simulink model "robot_segway_bloques"  (R2023b)
settings: Solver=ode15s  StartTime=0.0  StopTime=tiempo_final  MaxStep=1e-3  RelTol=1e-5  AbsTol=1e-7
values from neighbouring files (symbols this model uses):
  par = parametros_simulink(P, C)    [cargar_workspace.m]    (also in construir_robot_bloques.m = -R f   (manual sec. 7)'; simular_ode.m)
  Ts = se.Ts    [robot_controlador.m]    (also in simular_ode.m = P.sens.Ts; simular_slx.m = P.sens.Ts)
undefined symbols (not defined in the file or in its folder): angulo_servo_inicial, encoders_iniciales, estados_iniciales, inclinacion_inicial_est, medidas_iniciales, retardo_muestras, semilla
libraries: simulink x10
(part 2 of 2)

== system robot_segway_bloques/Robot/Servo y pata ==
  note: Servo PD sobre theta(l) con limite par-velocidad, F_l = n_servos tau dtheta/dl ; topes de carrera ; flexor opcional en serie (l_mec) (manual sec. 5 y 8)
  comandos : Inport
  cuerpo : Inport  Port=2
  1 entre m mecanismo : Gain  Gain=1/par.pata.masa_mecanismo
  Flexor (resorte en serie) : Subsystem
  Servo (PD con limite par-velocidad) : Subsystem
  Topes de carrera : Subsystem
  acel mec (si flexor) : Switch  Criteria=u2 > Threshold  Threshold=0.5  SaturateOnIntegerOverflow=off  InputSameDT=off
  amortiguamiento de pata b_pata : Gain  Gain=par.cuerpo.amort_pata
  amortiguamiento del mecanismo : Gain  Gain=par.cuerpo.amort_pata
  bus pata : BusCreator  Inputs=5
  cero : Constant  Value=0
  consigna : BusSelector  OutputSignals=angulo_servo_ref
  d largo mec (si flexor) : Switch  Criteria=u2 > Threshold  Threshold=0.5  SaturateOnIntegerOverflow=off  InputSameDT=off
  flexor activo : Constant  Value=par.pata.flexor_activo
  fuerza sobre l : Switch  Criteria=u2 > Threshold  Threshold=0.5  SaturateOnIntegerOverflow=off  InputSameDT=off
  integrador largo mecanismo : Integrator  InitialCondition=estados_iniciales(19)
  integrador vel mecanismo : Integrator  InitialCondition=estados_iniciales(20)
  largo de pata : BusSelector  OutputSignals=largo_pata,d_largo_pata
  largo que mueve el servo : Switch  Criteria=u2 > Threshold  Threshold=0.5  SaturateOnIntegerOverflow=off  InputSameDT=off
  servo + topes - amort : Sum  Inputs=++-
  servo - flexor + topes - amort : Sum  Inputs=+-+-
  velocidad que ve el servo : Switch  Criteria=u2 > Threshold  Threshold=0.5  SaturateOnIntegerOverflow=off  InputSameDT=off
  pata : Outport
  wires:
  comandos/1 -> consigna/1
  cuerpo/1 -> largo de pata/1
  integrador vel mecanismo/1 -> d largo mec (si flexor)/1, velocidad que ve el servo/1, Flexor (resorte en serie)/3(d_largo_mecanismo), amortiguamiento del mecanismo/1, bus pata/5  "d_largo_mecanismo"
  flexor activo/1 -> d largo mec (si flexor)/2, acel mec (si flexor)/2, largo que mueve el servo/2, velocidad que ve el servo/2, fuerza sobre l/2
  cero/1 -> d largo mec (si flexor)/3, acel mec (si flexor)/3
  d largo mec (si flexor)/1 -> integrador largo mecanismo/1
  acel mec (si flexor)/1 -> integrador vel mecanismo/1
  integrador largo mecanismo/1 -> largo que mueve el servo/1, Flexor (resorte en serie)/1(largo_mecanismo), bus pata/4  "largo_mecanismo"
  largo de pata/1 -> largo que mueve el servo/3, Flexor (resorte en serie)/2(largo_pata)  "<largo_pata>"
  largo de pata/2 -> velocidad que ve el servo/3, Flexor (resorte en serie)/4(d_largo_pata), amortiguamiento de pata b_pata/1  "<d_largo_pata>"
  consigna/1 -> Servo (PD con limite par-velocidad)/1(angulo_ref)  "<angulo_servo_ref>"
  largo que mueve el servo/1 -> Servo (PD con limite par-velocidad)/2(largo), Topes de carrera/1(largo)  "largo_q"
  velocidad que ve el servo/1 -> Servo (PD con limite par-velocidad)/3(d_largo), Topes de carrera/2(d_largo)  "d_largo_q"
  Servo (PD con limite par-velocidad)/3(fuerza_servo) -> servo + topes - amort/1, servo - flexor + topes - amort/1  "fuerza_servo"
  Topes de carrera/1(fuerza_tope) -> servo + topes - amort/2, servo - flexor + topes - amort/3  "fuerza_topes"
  amortiguamiento de pata b_pata/1 -> servo + topes - amort/3
  Flexor (resorte en serie)/1(fuerza_flexor) -> fuerza sobre l/1, servo - flexor + topes - amort/2  "fuerza_flexor"
  servo + topes - amort/1 -> fuerza sobre l/3
  amortiguamiento del mecanismo/1 -> servo - flexor + topes - amort/4
  servo - flexor + topes - amort/1 -> 1 entre m mecanismo/1
  1 entre m mecanismo/1 -> acel mec (si flexor)/1
  fuerza sobre l/1 -> bus pata/1  "fuerza_pata"
  Servo (PD con limite par-velocidad)/1(par_servo) -> bus pata/2  "par_servo"
  Servo (PD con limite par-velocidad)/2(angulo_servo) -> bus pata/3  "angulo_servo"
  bus pata/1 -> pata/1

== system robot_segway_bloques/Sensores/Acelerometro ==
  f_x : Inport
  f_y : Inport  Port=2
  f_x + ruido : Sum
  f_y + ruido : Sum
  rms del ruido x : Gain  Gain=par.sensores.acel_ruido
  rms del ruido y : Gain  Gain=par.sensores.acel_ruido
  ruido eje x : RandomNumber  Seed=semilla+1  SampleTime=Ts
  ruido eje y : RandomNumber  Seed=semilla+2  SampleTime=Ts
  acel_x : Outport
  acel_y : Outport  Port=2
  wires:
  rms del ruido y/1 -> f_y + ruido/2
  ruido eje y/1 -> rms del ruido y/1
  ruido eje x/1 -> rms del ruido x/1
  f_y/1 -> f_y + ruido/1
  f_x/1 -> f_x + ruido/1
  f_y + ruido/1 -> acel_y/1
  f_x + ruido/1 -> acel_x/1
  rms del ruido x/1 -> f_x + ruido/2

== system robot_segway_bloques/Sensores/Encoders ==
  ang_izq : Inport
  ang_der : Inport  Port=2
  cuenta entera der : Rounding
  cuenta entera izq : Rounding
  cuentas por radian der : Gain  Gain=par.sensores.CPR/(2*pi)
  cuentas por radian izq : Gain  Gain=par.sensores.CPR/(2*pi)
  encoder habilitado : Constant  Value=par.sensores.encoder
  si hay encoder der : Switch  Criteria=u2 > Threshold  Threshold=0.5  SaturateOnIntegerOverflow=off  InputSameDT=off
  si hay encoder izq : Switch  Criteria=u2 > Threshold  Threshold=0.5  SaturateOnIntegerOverflow=off  InputSameDT=off
  sin encoder (NaN) : Constant  Value=NaN
  encoder_izq : Outport
  encoder_der : Outport  Port=2
  wires:
  cuentas por radian der/1 -> cuenta entera der/1
  cuenta entera der/1 -> si hay encoder der/1
  encoder habilitado/1 -> si hay encoder izq/2, si hay encoder der/2
  ang_izq/1 -> cuentas por radian izq/1
  cuenta entera izq/1 -> si hay encoder izq/1
  ang_der/1 -> cuentas por radian der/1
  cuentas por radian izq/1 -> cuenta entera izq/1
  si hay encoder der/1 -> encoder_der/1
  sin encoder (NaN)/1 -> si hay encoder izq/3, si hay encoder der/3
  si hay encoder izq/1 -> encoder_izq/1

== system robot_segway_bloques/Sensores/Giroscopio ==
  vel_cabeceo : Inport
  giro + sesgo + ruido : Sum  Inputs=+++
  rms del ruido : Gain  Gain=par.sensores.gyro_ruido
  ruido blanco : RandomNumber  Seed=semilla  SampleTime=Ts
  saturacion del giroscopo : Saturate  UpperLimit=par.sensores.gyro_sat  LowerLimit=-par.sensores.gyro_sat
  sesgo : Constant  Value=par.sensores.gyro_sesgo
  giroscopo : Outport
  wires:
  ruido blanco/1 -> rms del ruido/1
  giro + sesgo + ruido/1 -> saturacion del giroscopo/1
  vel_cabeceo/1 -> giro + sesgo + ruido/1
  sesgo/1 -> giro + sesgo + ruido/2
  saturacion del giroscopo/1 -> giroscopo/1
  rms del ruido/1 -> giro + sesgo + ruido/3  "ruido"

== system robot_segway_bloques/Robot/Contacto rueda-piso/Friccion rueda derecha ==
  deslizamiento : Inport
  normal_por_rueda : Inport  Port=2
  mu : Inport  Port=3
  contacto : Inport  Port=4
  1 entre v0 : Gain  Gain=1/par.rueda.v0
  Coulomb - viscosa : Sum  Inputs=+-
  mu N tanh : Product  Inputs=***
  solo con contacto : Product  Inputs=**
  tanh : Trigonometry  Operator=tanh
  viscosa c_v : Gain  Gain=par.rueda.c_v
  fuerza : Outport
  wires:
  deslizamiento/1 -> viscosa c_v/1, 1 entre v0/1
  Coulomb - viscosa/1 -> solo con contacto/1
  mu N tanh/1 -> Coulomb - viscosa/1
  tanh/1 -> mu N tanh/3
  normal_por_rueda/1 -> mu N tanh/2
  1 entre v0/1 -> tanh/1
  mu/1 -> mu N tanh/1
  viscosa c_v/1 -> Coulomb - viscosa/2
  contacto/1 -> solo con contacto/2
  solo con contacto/1 -> fuerza/1

== system robot_segway_bloques/Robot/Contacto rueda-piso/Friccion rueda izquierda ==
  deslizamiento : Inport
  normal_por_rueda : Inport  Port=2
  mu : Inport  Port=3
  contacto : Inport  Port=4
  1 entre v0 : Gain  Gain=1/par.rueda.v0
  Coulomb - viscosa : Sum  Inputs=+-
  mu N tanh : Product  Inputs=***
  solo con contacto : Product  Inputs=**
  tanh : Trigonometry  Operator=tanh
  viscosa c_v : Gain  Gain=par.rueda.c_v
  fuerza : Outport
  wires:
  Coulomb - viscosa/1 -> solo con contacto/1
  mu/1 -> mu N tanh/1
  deslizamiento/1 -> viscosa c_v/1, 1 entre v0/1
  normal_por_rueda/1 -> mu N tanh/2
  1 entre v0/1 -> tanh/1
  tanh/1 -> mu N tanh/3
  mu N tanh/1 -> Coulomb - viscosa/1
  viscosa c_v/1 -> Coulomb - viscosa/2
  contacto/1 -> solo con contacto/2
  solo con contacto/1 -> fuerza/1

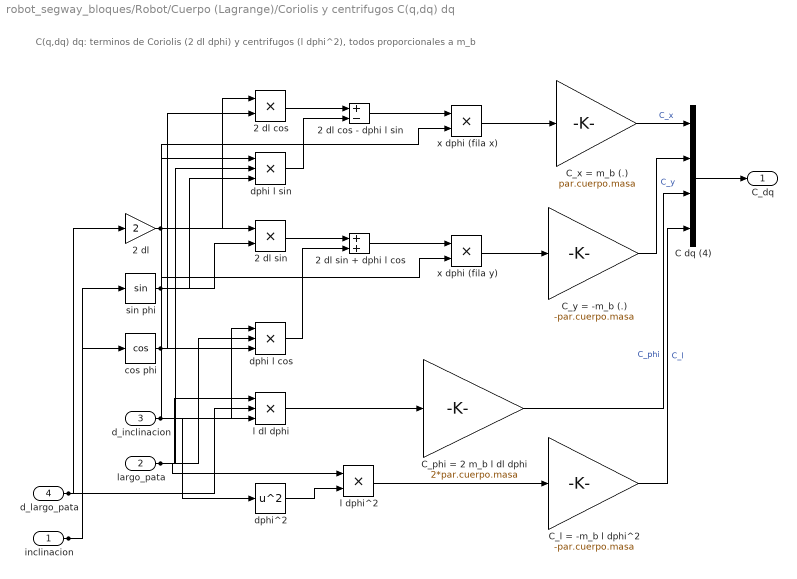
== system robot_segway_bloques/Robot/Cuerpo (Lagrange)/Coriolis y centrifugos C(q,dq) dq ==
  note: C(q,dq) dq: terminos de Coriolis (2 dl dphi) y centrifugos (l dphi^2), todos proporcionales a m_b
  inclinacion : Inport
  largo_pata : Inport  Port=2
  d_inclinacion : Inport  Port=3
  d_largo_pata : Inport  Port=4
  2 dl : Gain  Gain=2
  2 dl cos : Product  Inputs=**
  2 dl cos - dphi l sin : Sum  Inputs=+-
  2 dl sin : Product  Inputs=**
  2 dl sin + dphi l cos : Sum
  C dq (4) : Mux
  C_l = -m_b l dphi^2 : Gain  Gain=-par.cuerpo.masa
  C_phi = 2 m_b l dl dphi : Gain  Gain=2*par.cuerpo.masa
  C_x = m_b (.) : Gain  Gain=par.cuerpo.masa
  C_y = -m_b (.) : Gain  Gain=-par.cuerpo.masa
  cos phi : Trigonometry  Operator=cos
  dphi l cos : Product  Inputs=***
  dphi l sin : Product  Inputs=***
  dphi^2 : Math  Operator=square
  l dl dphi : Product  Inputs=***
  l dphi^2 : Product  Inputs=**
  sin phi : Trigonometry
  x dphi (fila x) : Product  Inputs=**
  x dphi (fila y) : Product  Inputs=**
  C_dq : Outport
  wires:
  largo_pata/1 -> l dphi^2/1, dphi l cos/2, dphi l sin/2, l dl dphi/1
  2 dl/1 -> 2 dl cos/1, 2 dl sin/1
  d_largo_pata/1 -> l dl dphi/2, 2 dl/1
  2 dl cos/1 -> 2 dl cos - dphi l sin/1
  d_inclinacion/1 -> x dphi (fila x)/2, x dphi (fila y)/2, l dl dphi/3, dphi l sin/1, dphi^2/1, dphi l cos/1
  inclinacion/1 -> sin phi/1, cos phi/1
  sin phi/1 -> 2 dl sin/2, dphi l sin/3
  cos phi/1 -> 2 dl cos/2, dphi l cos/3
  dphi l sin/1 -> 2 dl cos - dphi l sin/2
  2 dl sin/1 -> 2 dl sin + dphi l cos/1
  dphi l cos/1 -> 2 dl sin + dphi l cos/2
  l dl dphi/1 -> C_phi = 2 m_b l dl dphi/1
  dphi^2/1 -> l dphi^2/2
  2 dl cos - dphi l sin/1 -> x dphi (fila x)/1
  2 dl sin + dphi l cos/1 -> x dphi (fila y)/1
  l dphi^2/1 -> C_l = -m_b l dphi^2/1
  x dphi (fila x)/1 -> C_x = m_b (.)/1
  x dphi (fila y)/1 -> C_y = -m_b (.)/1
  C_phi = 2 m_b l dl dphi/1 -> C dq (4)/3  "C_phi"
  C_x = m_b (.)/1 -> C dq (4)/1  "C_x"
  C_y = -m_b (.)/1 -> C dq (4)/2  "C_y"
  C_l = -m_b l dphi^2/1 -> C dq (4)/4  "C_l"
  C dq (4)/1 -> C_dq/1

== system robot_segway_bloques/Robot/Cuerpo (Lagrange)/Fuerzas generalizadas Q ==
  note: Q por trabajo virtual (manual sec. 5): contacto, empuje F_x, pares de rueda con reaccion sobre el cuerpo, momento M_p, fuerza de la pata
  fuerza_contacto_x : Inport
  fuerza_contacto_y : Inport  Port=2
  par_reductor_izq : Inport  Port=3
  par_reductor_der : Inport  Port=4
  fuerza_pata : Inport  Port=5
  F_x : Inport  Port=6
  M_p : Inport  Port=7
  F_escalon : Inport  Port=8
  inclinacion : Inport  Port=9
  largo_pata : Inport  Port=10
  d_inclinacion : Inport  Port=11
  F_x l cos phi : Product  Inputs=***
  F_x sin phi : Product  Inputs=**
  Q = [Q_x; Q_y; Q_phi; Q_l] : Mux
  Q_l = fuerza_pata + F_x sin : Sum
  Q_phi = -tau_izq - tau_der + M_p + F_x l cos - b dphi : Sum  Inputs=--++-
  Q_x = F_cx + F_x + F_esc : Sum  Inputs=+++
  amortiguamiento de cabeceo : Gain  Gain=par.cuerpo.amort_cabeceo
  cos phi : Trigonometry  Operator=cos
  sin phi : Trigonometry
  Q : Outport
  wires:
  amortiguamiento de cabeceo/1 -> Q_phi = -tau_izq - tau_der + M_p + F_x l cos - b dphi/5
  d_inclinacion/1 -> amortiguamiento de cabeceo/1
  Q = [Q_x; Q_y; Q_phi; Q_l]/1 -> Q/1
  inclinacion/1 -> sin phi/1, cos phi/1
  fuerza_contacto_x/1 -> Q_x = F_cx + F_x + F_esc/1
  F_x sin phi/1 -> Q_l = fuerza_pata + F_x sin/2
  sin phi/1 -> F_x sin phi/2
  cos phi/1 -> F_x l cos phi/3
  largo_pata/1 -> F_x l cos phi/2
  F_escalon/1 -> Q_x = F_cx + F_x + F_esc/3
  F_x/1 -> Q_x = F_cx + F_x + F_esc/2, F_x l cos phi/1, F_x sin phi/1
  Q_x = F_cx + F_x + F_esc/1 -> Q = [Q_x; Q_y; Q_phi; Q_l]/1  "Q_x"
  par_reductor_izq/1 -> Q_phi = -tau_izq - tau_der + M_p + F_x l cos - b dphi/1
  par_reductor_der/1 -> Q_phi = -tau_izq - tau_der + M_p + F_x l cos - b dphi/2
  M_p/1 -> Q_phi = -tau_izq - tau_der + M_p + F_x l cos - b dphi/3
  F_x l cos phi/1 -> Q_phi = -tau_izq - tau_der + M_p + F_x l cos - b dphi/4
  fuerza_pata/1 -> Q_l = fuerza_pata + F_x sin/1
  fuerza_contacto_y/1 -> Q = [Q_x; Q_y; Q_phi; Q_l]/2  "Q_y"
  Q_phi = -tau_izq - tau_der + M_p + F_x l cos - b dphi/1 -> Q = [Q_x; Q_y; Q_phi; Q_l]/3  "Q_phi"
  Q_l = fuerza_pata + F_x sin/1 -> Q = [Q_x; Q_y; Q_phi; Q_l]/4  "Q_l"

== system robot_segway_bloques/Robot/Cuerpo (Lagrange)/Gravedad G(q) ==
  note: G(q): gravedad rotada por la pendiente alpha del piso (alpha = 0 en piso horizontal)
  inclinacion : Inport
  largo_pata : Inport  Port=2
  pendiente : Inport  Port=3
  G (4) : Mux
  G_l = g m_b cos(alpha - phi) : Gain  Gain=par.g*par.cuerpo.masa
  G_phi = g m_b l sin(alpha - phi) : Gain  Gain=par.g*par.cuerpo.masa
  G_x = g m_t sin alpha : Gain  Gain=par.g*(par.cuerpo.masa + par.rueda.masa_eje)
  G_y = g m_t cos alpha : Gain  Gain=par.g*(par.cuerpo.masa + par.rueda.masa_eje)
  alpha - phi : Sum  Inputs=+-
  cos alpha : Trigonometry  Operator=cos
  cos(alpha - phi) : Trigonometry  Operator=cos
  l sin(alpha - phi) : Product  Inputs=**
  sin alpha : Trigonometry
  sin(alpha - phi) : Trigonometry
  G : Outport
  wires:
  inclinacion/1 -> alpha - phi/2
  pendiente/1 -> cos alpha/1, sin alpha/1, alpha - phi/1
  cos(alpha - phi)/1 -> G_l = g m_b cos(alpha - phi)/1
  sin alpha/1 -> G_x = g m_t sin alpha/1
  alpha - phi/1 -> sin(alpha - phi)/1, cos(alpha - phi)/1
  cos alpha/1 -> G_y = g m_t cos alpha/1
  largo_pata/1 -> l sin(alpha - phi)/1
  sin(alpha - phi)/1 -> l sin(alpha - phi)/2
  G_x = g m_t sin alpha/1 -> G (4)/1  "G_x"
  G_y = g m_t cos alpha/1 -> G (4)/2  "G_y"
  l sin(alpha - phi)/1 -> G_phi = g m_b l sin(alpha - phi)/1
  G_phi = g m_b l sin(alpha - phi)/1 -> G (4)/3  "G_phi"
  G_l = g m_b cos(alpha - phi)/1 -> G (4)/4  "G_l"
  G (4)/1 -> G/1

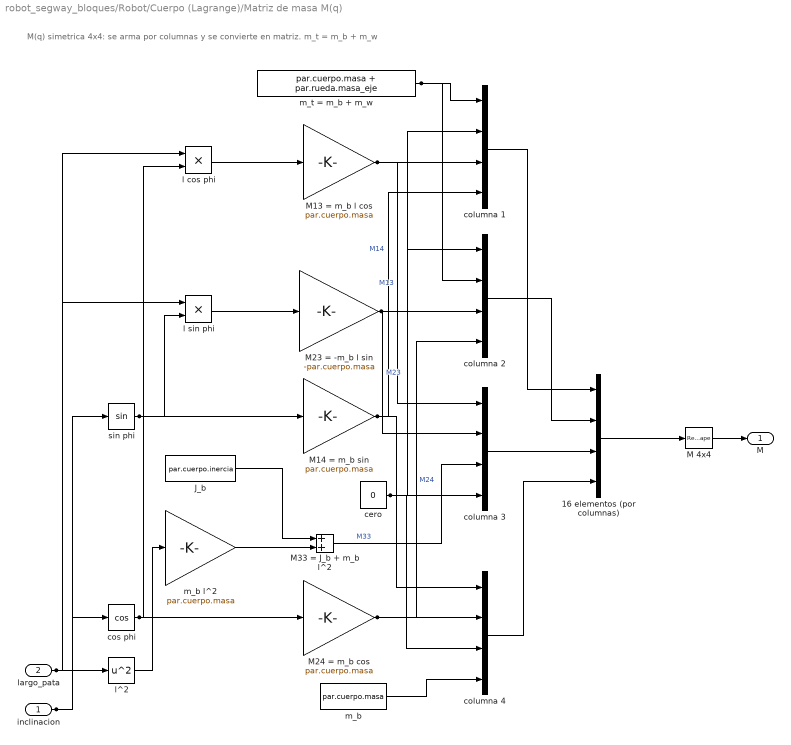
== system robot_segway_bloques/Robot/Cuerpo (Lagrange)/Matriz de masa M(q) ==
  note: M(q) simetrica 4x4: se arma por columnas y se convierte en matriz. m_t = m_b + m_w
  inclinacion : Inport
  largo_pata : Inport  Port=2
  16 elementos (por columnas) : Mux
  J_b : Constant  Value=par.cuerpo.inercia
  M 4x4 : Reshape  OutputDimensionality=Customize  OutputDimensions=[4 4]
  M13 = m_b l cos : Gain  Gain=par.cuerpo.masa
  M14 = m_b sin : Gain  Gain=par.cuerpo.masa
  M23 = -m_b l sin : Gain  Gain=-par.cuerpo.masa
  M24 = m_b cos : Gain  Gain=par.cuerpo.masa
  M33 = J_b + m_b l^2 : Sum
  cero : Constant  Value=0
  columna {1..4} (4 alike) : Mux
  cos phi : Trigonometry  Operator=cos
  l cos phi : Product  Inputs=**
  l sin phi : Product  Inputs=**
  l^2 : Math  Operator=square
  m_b : Constant  Value=par.cuerpo.masa
  m_b l^2 : Gain  Gain=par.cuerpo.masa
  m_t = m_b + m_w : Constant  Value=par.cuerpo.masa + par.rueda.masa_eje
  sin phi : Trigonometry
  M : Outport
  wires:
  largo_pata/1 -> l cos phi/1, l sin phi/1, l^2/1
  l cos phi/1 -> M13 = m_b l cos/1
  inclinacion/1 -> cos phi/1, sin phi/1
  l sin phi/1 -> M23 = -m_b l sin/1
  sin phi/1 -> M14 = m_b sin/1, l sin phi/2
  l^2/1 -> m_b l^2/1
  cos phi/1 -> l cos phi/2, M24 = m_b cos/1
  cero/1 -> columna 1/2, columna 2/1, columna 3/4, columna 4/3
  J_b/1 -> M33 = J_b + m_b l^2/1
  m_b l^2/1 -> M33 = J_b + m_b l^2/2
  m_t = m_b + m_w/1 -> columna 1/1, columna 2/2
  M33 = J_b + m_b l^2/1 -> columna 3/3  "M33"
  M13 = m_b l cos/1 -> columna 1/3, columna 3/1  "M13"
  M23 = -m_b l sin/1 -> columna 2/3, columna 3/2  "M23"
  M14 = m_b sin/1 -> columna 1/4, columna 4/1  "M14"
  M24 = m_b cos/1 -> columna 2/4, columna 4/2  "M24"
  m_b/1 -> columna 4/4
  columna 1/1 -> 16 elementos (por columnas)/1
  columna 2/1 -> 16 elementos (por columnas)/2
  columna 3/1 -> 16 elementos (por columnas)/3
  columna 4/1 -> 16 elementos (por columnas)/4
  16 elementos (por columnas)/1 -> M 4x4/1
  M 4x4/1 -> M/1

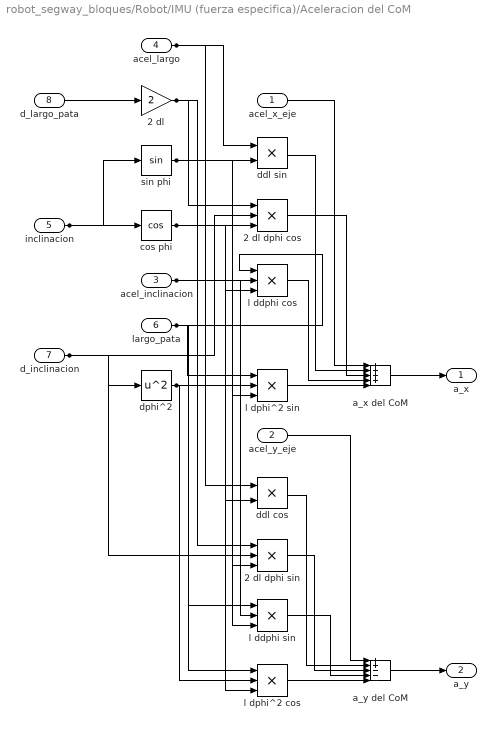
== system robot_segway_bloques/Robot/IMU (fuerza especifica)/Aceleracion del CoM ==
  acel_x_eje : Inport
  acel_y_eje : Inport  Port=2
  acel_inclinacion : Inport  Port=3
  acel_largo : Inport  Port=4
  inclinacion : Inport  Port=5
  largo_pata : Inport  Port=6
  d_inclinacion : Inport  Port=7
  d_largo_pata : Inport  Port=8
  2 dl : Gain  Gain=2
  2 dl dphi cos : Product  Inputs=***
  2 dl dphi sin : Product  Inputs=***
  a_x del CoM : Sum  Inputs=++++-
  a_y del CoM : Sum  Inputs=++---
  cos phi : Trigonometry  Operator=cos
  ddl cos : Product  Inputs=**
  ddl sin : Product  Inputs=**
  dphi^2 : Math  Operator=square
  l ddphi cos : Product  Inputs=***
  l ddphi sin : Product  Inputs=***
  l dphi^2 cos : Product  Inputs=***
  l dphi^2 sin : Product  Inputs=***
  sin phi : Trigonometry
  a_x : Outport
  a_y : Outport  Port=2
  wires:
  2 dl/1 -> 2 dl dphi cos/1, 2 dl dphi sin/1
  acel_inclinacion/1 -> l ddphi cos/2, l ddphi sin/2
  acel_x_eje/1 -> a_x del CoM/1
  acel_largo/1 -> ddl sin/1, ddl cos/1
  d_largo_pata/1 -> 2 dl/1
  d_inclinacion/1 -> 2 dl dphi cos/2, 2 dl dphi sin/2, dphi^2/1
  inclinacion/1 -> cos phi/1, sin phi/1
  sin phi/1 -> 2 dl dphi sin/3, ddl sin/2, l ddphi sin/3, l dphi^2 sin/3
  cos phi/1 -> ddl cos/2, 2 dl dphi cos/3, l ddphi cos/3, l dphi^2 cos/3
  largo_pata/1 -> l ddphi cos/1, l dphi^2 sin/1, l dphi^2 cos/1, l ddphi sin/1
  dphi^2/1 -> l dphi^2 sin/2, l dphi^2 cos/2
  ddl sin/1 -> a_x del CoM/2
  2 dl dphi cos/1 -> a_x del CoM/3
  l ddphi cos/1 -> a_x del CoM/4
  l dphi^2 sin/1 -> a_x del CoM/5
  acel_y_eje/1 -> a_y del CoM/1
  ddl cos/1 -> a_y del CoM/2
  a_x del CoM/1 -> a_x/1
  2 dl dphi sin/1 -> a_y del CoM/3
  l ddphi sin/1 -> a_y del CoM/4
  l dphi^2 cos/1 -> a_y del CoM/5
  a_y del CoM/1 -> a_y/1

== system robot_segway_bloques/Robot/IMU (fuerza especifica)/Aceleracion en el punto de la IMU ==
  a_com_x : Inport
  a_com_y : Inport  Port=2
  inclinacion : Inport  Port=3
  d_inclinacion : Inport  Port=4
  acel_inclinacion : Inport  Port=5
  a_imu_x = a_x + ddphi dw_y - dphi^2 dw_x : Sum  Inputs=++-
  a_imu_y = a_y - ddphi dw_x - dphi^2 dw_y : Sum  Inputs=+--
  cos phi : Trigonometry  Operator=cos
  d_ix cos : Gain  Gain=par.sensores.imu_dx
  d_ix sin : Gain  Gain=par.sensores.imu_dx
  d_iy cos : Gain  Gain=par.sensores.imu_dy
  d_iy sin : Gain  Gain=par.sensores.imu_dy
  ddphi dw_x : Product  Inputs=**
  ddphi dw_y : Product  Inputs=**
  dphi^2 : Math  Operator=square
  dphi^2 dw_x : Product  Inputs=**
  dphi^2 dw_y : Product  Inputs=**
  dw_x = d_ix cos + d_iy sin : Sum
  dw_y = -d_ix sin + d_iy cos : Sum  Inputs=-+
  sin phi : Trigonometry
  a_imu_x : Outport
  a_imu_y : Outport  Port=2
  wires:
  ddphi dw_y/1 -> a_imu_x = a_x + ddphi dw_y - dphi^2 dw_x/2
  acel_inclinacion/1 -> ddphi dw_y/1, ddphi dw_x/1
  sin phi/1 -> d_iy sin/1, d_ix sin/1
  inclinacion/1 -> cos phi/1, sin phi/1
  d_iy sin/1 -> dw_x = d_ix cos + d_iy sin/2
  d_inclinacion/1 -> dphi^2/1
  d_ix cos/1 -> dw_x = d_ix cos + d_iy sin/1
  a_imu_x = a_x + ddphi dw_y - dphi^2 dw_x/1 -> a_imu_x/1
  dphi^2 dw_x/1 -> a_imu_x = a_x + ddphi dw_y - dphi^2 dw_x/3
  d_iy cos/1 -> dw_y = -d_ix sin + d_iy cos/2
  d_ix sin/1 -> dw_y = -d_ix sin + d_iy cos/1
  cos phi/1 -> d_ix cos/1, d_iy cos/1
  dphi^2/1 -> dphi^2 dw_x/1, dphi^2 dw_y/1
  dw_y = -d_ix sin + d_iy cos/1 -> dphi^2 dw_y/2, ddphi dw_y/2  "dw_y"
  dw_x = d_ix cos + d_iy sin/1 -> ddphi dw_x/2, dphi^2 dw_x/2  "dw_x"
  a_imu_y = a_y - ddphi dw_x - dphi^2 dw_y/1 -> a_imu_y/1
  a_com_y/1 -> a_imu_y = a_y - ddphi dw_x - dphi^2 dw_y/1
  a_com_x/1 -> a_imu_x = a_x + ddphi dw_y - dphi^2 dw_x/1
  dphi^2 dw_y/1 -> a_imu_y = a_y - ddphi dw_x - dphi^2 dw_y/3
  ddphi dw_x/1 -> a_imu_y = a_y - ddphi dw_x - dphi^2 dw_y/2

== system robot_segway_bloques/Robot/IMU (fuerza especifica)/Fuerza especifica en marco cuerpo ==
  a_imu_x : Inport
  a_imu_y : Inport  Port=2
  inclinacion : Inport  Port=3
  pendiente : Inport  Port=4
  cos alpha : Trigonometry  Operator=cos
  cos f_x : Product  Inputs=**
  cos f_y : Product  Inputs=**
  cos phi : Trigonometry  Operator=cos
  f_x piso = a_x + g sin alpha : Sum
  f_y piso = a_y + g cos alpha : Sum
  fb_x = cos f_x - sin f_y : Sum  Inputs=+-
  fb_y = sin f_x + cos f_y : Sum
  g cos alpha : Gain  Gain=par.g
  g sin alpha : Gain  Gain=par.g
  sin alpha : Trigonometry
  sin f_x : Product  Inputs=**
  sin f_y : Product  Inputs=**
  sin phi : Trigonometry
  fb_x : Outport
  fb_y : Outport  Port=2
  wires:
  fb_x = cos f_x - sin f_y/1 -> fb_x/1
  cos f_y/1 -> fb_y = sin f_x + cos f_y/2
  sin f_x/1 -> fb_y = sin f_x + cos f_y/1
  a_imu_y/1 -> f_y piso = a_y + g cos alpha/1
  cos alpha/1 -> g cos alpha/1
  pendiente/1 -> cos alpha/1, sin alpha/1
  g cos alpha/1 -> f_y piso = a_y + g cos alpha/2
  sin phi/1 -> sin f_y/1, sin f_x/1
  inclinacion/1 -> cos phi/1, sin phi/1
  g sin alpha/1 -> f_x piso = a_x + g sin alpha/2
  a_imu_x/1 -> f_x piso = a_x + g sin alpha/1
  cos f_x/1 -> fb_x = cos f_x - sin f_y/1
  sin alpha/1 -> g sin alpha/1
  f_x piso = a_x + g sin alpha/1 -> cos f_x/2, sin f_x/2  "f_x_piso"
  fb_y = sin f_x + cos f_y/1 -> fb_y/1
  cos phi/1 -> cos f_x/1, cos f_y/1
  f_y piso = a_y + g cos alpha/1 -> sin f_y/2, cos f_y/2  "f_y_piso"
  sin f_y/1 -> fb_x = cos f_x - sin f_y/2

== system robot_segway_bloques/Robot/Motores y reductores/Motor y reductor derecho ==
  tension : Inport
  vel_rueda : Inport  Port=2
  1 entre L : Gain  Gain=1/par.motor.L
  Coulomb tau_c : Gain  Gain=par.motor.tau_coulomb
  V - R i - fcem : Sum  Inputs=+--
  caida R i : Gain  Gain=par.motor.R
  fcem Ke w : Gain  Gain=par.motor.Ke
  friccion del rotor : Sum
  integrador de corriente : Integrator  InitialCondition=estados_iniciales(18)
  par electrico Kt i : Gain  Gain=par.motor.Kt
  par neto en el rotor : Sum  Inputs=+-
  reductor x N : Gain  Gain=par.motor.relacion
  relacion N : Gain  Gain=par.motor.relacion
  tanh : Trigonometry  Operator=tanh
  viscosa b_rotor : Gain  Gain=par.motor.b_rotor
  w entre 0.5 : Gain  Gain=2
  par_reductor : Outport
  corriente : Outport  Port=2
  wires:
  w entre 0.5/1 -> tanh/1
  vel_rueda/1 -> relacion N/1
  tanh/1 -> Coulomb tau_c/1
  integrador de corriente/1 -> caida R i/1, corriente/1, par electrico Kt i/1  "corriente"
  relacion N/1 -> viscosa b_rotor/1, w entre 0.5/1, fcem Ke w/1  "vel_rotor"
  fcem Ke w/1 -> V - R i - fcem/3  "fcem"
  V - R i - fcem/1 -> 1 entre L/1
  caida R i/1 -> V - R i - fcem/2
  tension/1 -> V - R i - fcem/1
  viscosa b_rotor/1 -> friccion del rotor/2
  1 entre L/1 -> integrador de corriente/1  "di_dt"
  Coulomb tau_c/1 -> friccion del rotor/1
  par electrico Kt i/1 -> par neto en el rotor/1  "par_electrico"
  friccion del rotor/1 -> par neto en el rotor/2  "friccion"
  par neto en el rotor/1 -> reductor x N/1
  reductor x N/1 -> par_reductor/1

== system robot_segway_bloques/Robot/Motores y reductores/Motor y reductor izquierdo ==
  tension : Inport
  vel_rueda : Inport  Port=2
  1 entre L : Gain  Gain=1/par.motor.L
  Coulomb tau_c : Gain  Gain=par.motor.tau_coulomb
  V - R i - fcem : Sum  Inputs=+--
  caida R i : Gain  Gain=par.motor.R
  fcem Ke w : Gain  Gain=par.motor.Ke
  friccion del rotor : Sum
  integrador de corriente : Integrator  InitialCondition=estados_iniciales(17)
  par electrico Kt i : Gain  Gain=par.motor.Kt
  par neto en el rotor : Sum  Inputs=+-
  reductor x N : Gain  Gain=par.motor.relacion
  relacion N : Gain  Gain=par.motor.relacion
  tanh : Trigonometry  Operator=tanh
  viscosa b_rotor : Gain  Gain=par.motor.b_rotor
  w entre 0.5 : Gain  Gain=2
  par_reductor : Outport
  corriente : Outport  Port=2
  wires:
  tension/1 -> V - R i - fcem/1
  Coulomb tau_c/1 -> friccion del rotor/1
  vel_rueda/1 -> relacion N/1
  fcem Ke w/1 -> V - R i - fcem/3  "fcem"
  relacion N/1 -> viscosa b_rotor/1, fcem Ke w/1, w entre 0.5/1  "vel_rotor"
  integrador de corriente/1 -> par electrico Kt i/1, corriente/1, caida R i/1  "corriente"
  V - R i - fcem/1 -> 1 entre L/1
  reductor x N/1 -> par_reductor/1
  caida R i/1 -> V - R i - fcem/2
  w entre 0.5/1 -> tanh/1
  tanh/1 -> Coulomb tau_c/1
  par electrico Kt i/1 -> par neto en el rotor/1  "par_electrico"
  viscosa b_rotor/1 -> friccion del rotor/2
  1 entre L/1 -> integrador de corriente/1  "di_dt"
  friccion del rotor/1 -> par neto en el rotor/2  "friccion"
  par neto en el rotor/1 -> reductor x N/1

== system robot_segway_bloques/Robot/Ruedas/Rueda derecha ==
  par_reductor : Inport
  par_contacto : Inport  Port=2
  1 entre J_eq (rueda + rotor reflejado) : Gain  Gain=1/(par.rueda.inercia + par.motor.relacion^2*par.motor.J_rotor)
  amortiguamiento b_w : Gain  Gain=par.rueda.amort
  integrador de angulo : Integrator  InitialCondition=estados_iniciales(11)
  integrador de velocidad : Integrator  InitialCondition=estados_iniciales(12)
  par neto : Sum  Inputs=++-
  ang_rueda : Outport
  vel_rueda : Outport  Port=2
  wires:
  par neto/1 -> 1 entre J_eq (rueda + rotor reflejado)/1
  par_contacto/1 -> par neto/2
  par_reductor/1 -> par neto/1
  integrador de angulo/1 -> ang_rueda/1  "ang_rueda"
  integrador de velocidad/1 -> amortiguamiento b_w/1, vel_rueda/1, integrador de angulo/1  "vel_rueda"
  1 entre J_eq (rueda + rotor reflejado)/1 -> integrador de velocidad/1  "acel_rueda"
  amortiguamiento b_w/1 -> par neto/3  "friccion"

== system robot_segway_bloques/Robot/Ruedas/Rueda izquierda ==
  par_reductor : Inport
  par_contacto : Inport  Port=2
  1 entre J_eq (rueda + rotor reflejado) : Gain  Gain=1/(par.rueda.inercia + par.motor.relacion^2*par.motor.J_rotor)
  amortiguamiento b_w : Gain  Gain=par.rueda.amort
  integrador de angulo : Integrator  InitialCondition=estados_iniciales(9)
  integrador de velocidad : Integrator  InitialCondition=estados_iniciales(10)
  par neto : Sum  Inputs=++-
  ang_rueda : Outport
  vel_rueda : Outport  Port=2
  wires:
  amortiguamiento b_w/1 -> par neto/3  "friccion"
  integrador de angulo/1 -> ang_rueda/1  "ang_rueda"
  integrador de velocidad/1 -> integrador de angulo/1, amortiguamiento b_w/1, vel_rueda/1  "vel_rueda"
  1 entre J_eq (rueda + rotor reflejado)/1 -> integrador de velocidad/1  "acel_rueda"
  par_contacto/1 -> par neto/2
  par_reductor/1 -> par neto/1
  par neto/1 -> 1 entre J_eq (rueda + rotor reflejado)/1

== system robot_segway_bloques/Robot/Servo y pata/Flexor (resorte en serie) ==
  largo_mecanismo : Inport
  largo_pata : Inport  Port=2
  d_largo_mecanismo : Inport  Port=3
  d_largo_pata : Inport  Port=4
  c flexor : Gain  Gain=par.pata.c_flexor
  c tope : Gain  Gain=par.cuerpo.c_tope
  compresion = l mec - l : Sum  Inputs=+-
  d compresion : Sum  Inputs=+-
  fuera de la carrera : DeadZone  LowerValue=0  UpperValue=par.pata.carrera_flexor
  fuerza del flexor : Sum  Inputs=++++
  k flexor : Gain  Gain=par.pata.k_flexor
  k tope : Gain  Gain=par.cuerpo.k_tope
  toca el tope : simulink/Logic and Bit Operations/Compare To Zero  relop=~=  OutDataTypeStr=boolean
  tope 0 o 1 : DataTypeConversion  OutDataTypeStr=double  SaturateOnIntegerOverflow=off  RndMeth=Floor
  vel si toca : Product  Inputs=**
  fuerza_flexor : Outport
  wires:
  d_largo_pata/1 -> d compresion/2
  c tope/1 -> fuerza del flexor/4
  compresion = l mec - l/1 -> k flexor/1, fuera de la carrera/1  "compresion"
  d_largo_mecanismo/1 -> d compresion/1
  fuera de la carrera/1 -> k tope/1, toca el tope/1  "exceso"
  largo_pata/1 -> compresion = l mec - l/2
  largo_mecanismo/1 -> compresion = l mec - l/1
  toca el tope/1 -> tope 0 o 1/1
  k flexor/1 -> fuerza del flexor/1
  d compresion/1 -> c flexor/1, vel si toca/2  "d_compresion"
  tope 0 o 1/1 -> vel si toca/1
  c flexor/1 -> fuerza del flexor/2
  vel si toca/1 -> c tope/1
  k tope/1 -> fuerza del flexor/3
  fuerza del flexor/1 -> fuerza_flexor/1

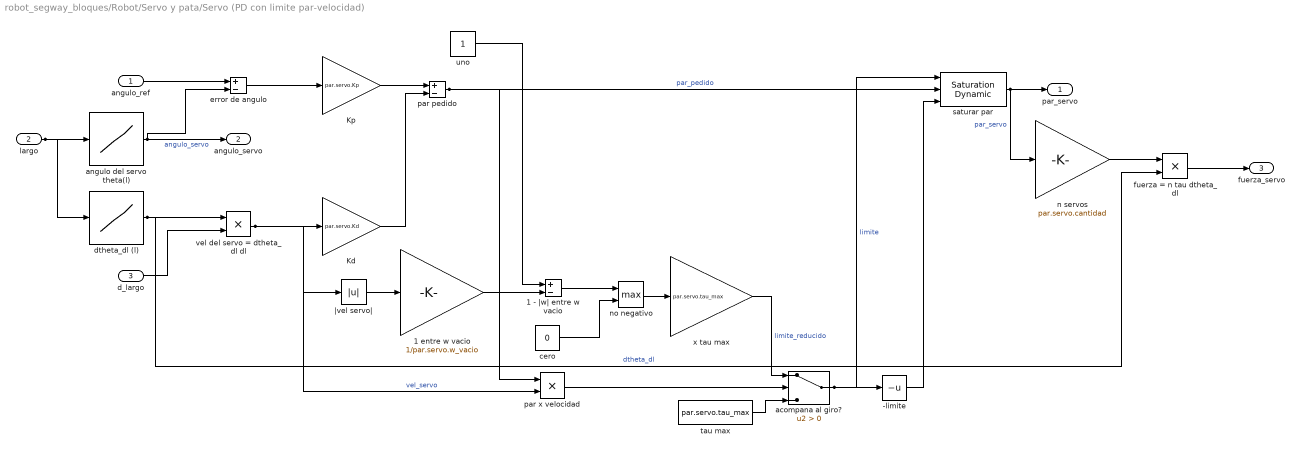
== system robot_segway_bloques/Robot/Servo y pata/Servo (PD con limite par-velocidad) ==
  angulo_ref : Inport
  largo : Inport  Port=2
  d_largo : Inport  Port=3
  -limite : UnaryMinus
  1 - |w| entre w vacio : Sum  Inputs=+-
  1 entre w vacio : Gain  Gain=1/par.servo.w_vacio
  Kd : Gain  Gain=par.servo.Kd
  Kp : Gain  Gain=par.servo.Kp
  acompana al giro? : Switch  Criteria=u2 > Threshold  SaturateOnIntegerOverflow=off  InputSameDT=off
  angulo del servo theta(l) : Lookup_n-D  NumberOfTableDimensions=1  BreakpointsForDimension1=par.pata.tabla_l  Table=par.pata.tabla_theta  InternalRulePriority=Speed  RndMeth=Simplest
  cero : Constant  Value=0
  dtheta_dl (l) : Lookup_n-D  NumberOfTableDimensions=1  BreakpointsForDimension1=par.pata.tabla_l  Table=par.pata.tabla_dtheta_dl  InternalRulePriority=Speed  RndMeth=Simplest
  error de angulo : Sum  Inputs=+-
  fuerza = n tau dtheta_dl : Product  Inputs=**
  n servos : Gain  Gain=par.servo.cantidad
  no negativo : MinMax  Function=max  Inputs=2
  par pedido : Sum  Inputs=+-
  par x velocidad : Product  Inputs=**
  saturar par : simulink/Discontinuities/Saturation Dynamic  OutMin=[]  OutMax=[]  OutDataTypeStr=Inherit: Same as second input  OutDataType=fixdt(1, 16)  OutScaling=2^-10  DoSatur=off
  tau max : Constant  Value=par.servo.tau_max
  uno : Constant
  vel del servo = dtheta_dl dl : Product  Inputs=**
  x tau max : Gain  Gain=par.servo.tau_max
  |vel servo| : Abs  SaturateOnIntegerOverflow=off
  par_servo : Outport
  angulo_servo : Outport  Port=2
  fuerza_servo : Outport  Port=3
  wires:
  error de angulo/1 -> Kp/1
  largo/1 -> angulo del servo theta(l)/1, dtheta_dl (l)/1
  uno/1 -> 1 - |w| entre w vacio/1
  d_largo/1 -> vel del servo = dtheta_dl dl/2
  angulo_ref/1 -> error de angulo/1
  tau max/1 -> acompana al giro?/3
  dtheta_dl (l)/1 -> fuerza = n tau dtheta_dl/2, vel del servo = dtheta_dl dl/1  "dtheta_dl"
  angulo del servo theta(l)/1 -> error de angulo/2, angulo_servo/1  "angulo_servo"
  vel del servo = dtheta_dl dl/1 -> par x velocidad/2, |vel servo|/1, Kd/1  "vel_servo"
  Kp/1 -> par pedido/1
  Kd/1 -> par pedido/2
  |vel servo|/1 -> 1 entre w vacio/1
  saturar par/1 -> par_servo/1, n servos/1  "par_servo"
  par pedido/1 -> saturar par/2, par x velocidad/1  "par_pedido"
  1 entre w vacio/1 -> 1 - |w| entre w vacio/2
  1 - |w| entre w vacio/1 -> no negativo/1
  cero/1 -> no negativo/2
  par x velocidad/1 -> acompana al giro?/2
  no negativo/1 -> x tau max/1
  x tau max/1 -> acompana al giro?/1  "limite_reducido"
  acompana al giro?/1 -> saturar par/1, -limite/1  "limite"
  -limite/1 -> saturar par/3
  n servos/1 -> fuerza = n tau dtheta_dl/1
  fuerza = n tau dtheta_dl/1 -> fuerza_servo/1

== system robot_segway_bloques/Robot/Servo y pata/Topes de carrera ==
  largo : Inport
  d_largo : Inport  Port=2
  -c tope : Gain  Gain=-par.cuerpo.c_tope
  -k tope : Gain  Gain=-par.cuerpo.k_tope
  cuanto se pasa del tope : DeadZone  LowerValue=par.pata.l_min  UpperValue=par.pata.l_max
  fuerza de tope : Sum
  toca el tope : simulink/Logic and Bit Operations/Compare To Zero  relop=~=  OutDataTypeStr=boolean
  tope 0 o 1 : DataTypeConversion  OutDataTypeStr=double  SaturateOnIntegerOverflow=off  RndMeth=Floor
  vel si toca : Product  Inputs=**
  fuerza_tope : Outport
  wires:
  -k tope/1 -> fuerza de tope/1
  fuerza de tope/1 -> fuerza_tope/1
  largo/1 -> cuanto se pasa del tope/1
  cuanto se pasa del tope/1 -> -k tope/1, toca el tope/1  "exceso"
  vel si toca/1 -> -c tope/1
  toca el tope/1 -> tope 0 o 1/1
  tope 0 o 1/1 -> vel si toca/1
  -c tope/1 -> fuerza de tope/2
  d_largo/1 -> vel si toca/2
